simulink model "MCHP_SMO_MCLV48V300W_dsPIC33CK64MC105_DIM"  (R2022b)
settings: Solver=FixedStepDiscrete  StartTime=0.0  StopTime=10.0  FixedStep=50e-6  RelTol=1e-3  EnableMultiTasking=on
undefined symbols (not defined in the file): A4, B0, C12, C13, C4, C5, C6, C8, C9, DiscIntNeverNeededParam, inverter, Iq_Ref_openLoop, Max, MaxPer, ms, NumBits1, NumBits2, P20, P32, P52, P53, P54, P56, P57, P60, P61, PI_params, Pin, pmsm, PU_System, PWM1max, PWM_frequency, Resol, s, Speed_Ref_openLoop, Ts, Ts_speed, us
libraries: simulink x30, MCHP_Blockset x18, mcbcontrolslib x9, slpidlib x3, mcbplantlib x1, autolibpmsmexterior x1
(part 1 of 4)
settings Model: ExtModeBatchMode=on  ExtModeEnableFloating=off  ExtModeTrigDuration=32  Creator=I67977  LastModifiedBy=I67977
settings OptimizationCC: DefaultParameterBehavior=Inlined  DefaultUnderspecifiedDataType=single  InlineInvariantSignals=on  EnhancedBackFolding=on  StrengthReduction=on  BooleansAsBitfields=on  PassReuseOutputArgsAs=Individual arguments  ZeroExternalMemoryAtStartup=off  ZeroInternalMemoryAtStartup=off  OptimizeBlockOrder=speed  DifferentSizesBufferReuse=on  EfficientTunableParamExpr=on
settings DebuggingCC: MultiTaskDSMMsg=none  MultiTaskCondExecSysMsg=none  MultiTaskRateTransMsg=warning  ParameterTunabilityLossMsg=error
settings HardwareCC: ProdBitPerInt=16  ProdBitPerPointer=16  ProdBitPerSizeT=16  ProdBitPerPtrDiffT=32  ProdLargestAtomicInteger=Integer  ProdLargestAtomicFloat=None  ProdWordSize=16  ProdLongLongMode=on  ProdHWDeviceType=Generic->Custom
settings ModelReferenceCC: ModelReferenceNumInstancesAllowed=Single
settings SFSimCC: MATLABDynamicMemAlloc=off
settings RTWCC: Description=Microchip Embedded Target PIC24 dsPIC30 dsPIC33 (real-time)  SystemTargetFile=MCHP_dsPIC_stf.tlc  TLCOptions="-aExtModeXCPClassicInterface=0  -aCreateExtModeTypes=1 -aExtModeXCPSimulationTimeInTicks=1"  TemplateMakefile=MCHP_dsPIC.tmf
settings CodeAppCC: ForceParamTrailComments=on  IgnoreCustomStorageClasses=off  MaxIdLength=255  OperatorAnnotations=on  SimulinkDataObjDesc=on  SFDataObjDesc=on  InsertBlockDesc=on
settings STFCustomTargetCC: TargetLibSuffix=_lib.a  CodeReplacementLibrary=Microchip Code Replacement Library for dsPIC  MultiwordLength=256  CombineOutputUpdateFcns=on  CombineSignalStateStructs=on  SuppressErrorStatus=on  ERTCustomFileBanners=on  SupportNonFinite=off  SupportContinuousTime=off  RemoveResetFunc=on  MATLABClassNameForMDSCustomization=Simulink.SoftwareTarget.ERTCustomization  SystemTargetFile=MCHP_dsPIC_stf.tlc
settings ERTTargetCC: TargetLibSuffix=_lib.a  CodeReplacementLibrary=Microchip Code Replacement Library for dsPIC  ParMdlRefBuildCompliant=off  CompOptLevelCompliant=off  ConcurrentExecutionCompliant=off  CombineSignalStateStructs=on  SuppressErrorStatus=on  SupportNonFinite=off  SupportNonInlinedSFcns=on  ModelStepFunctionPrototypeControlCompliant=off  CPPClassGenCompliant=off  UseToolchainInfoCompliant=off  ExtModeTransport=1  ExtModeStaticAlloc=on  ExtModeAutomaticAllocSize=off  ExtModeStaticAllocSize=2048  ExtModeMexFile=ext_xcp  ExtModeMexArgs=1 0 4000000 './MCHP_LVMC_template.X/MCHP_LVMC_template.elf'  ExtModeIntrfLevel=Level2 - Open  InlinedParameterPlacement=NonHierarchical  ERTSrcFileBannerTemplate=MCHP_dsPIC_code_template.cgt  ERTHdrFileBannerTemplate=MCHP_dsPIC_code_template.cgt  ERTDataSrcFileTemplate=MCHP_dsPIC_code_template.cgt  ERTDataHdrFileTemplate=MCHP_dsPIC_code_template.cgt  ERTCustomFileTemplate=MCHP_main.tlc  MaxLineWidth=110

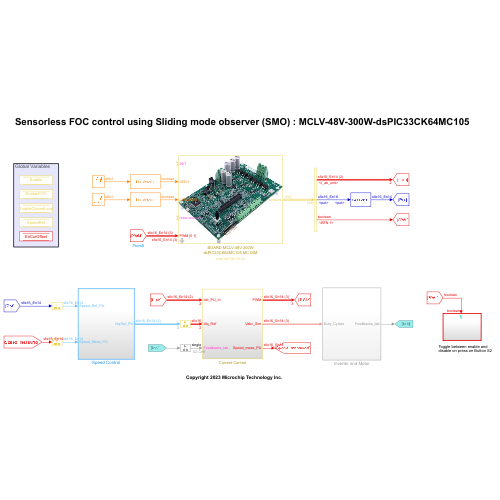
[thumbnail: Simulink's stored preview of the top-level diagram]
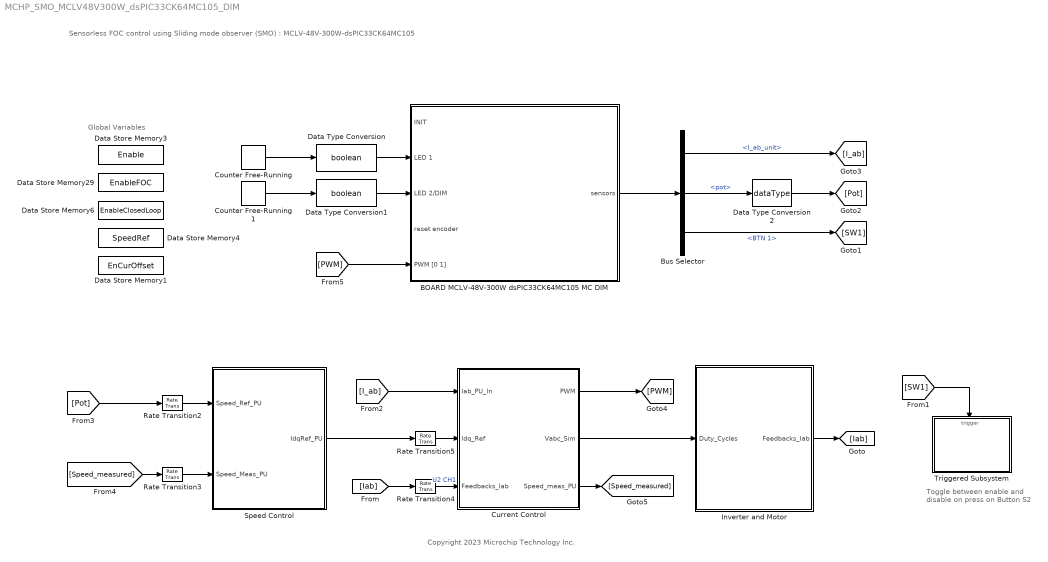
== system MCHP_SMO_MCLV48V300W_dsPIC33CK64MC105_DIM ==
  note: Toggle between enable and disable on press on Button S2
  note: Copyright 2023 Microchip Technology Inc.
  note: Global Variables
  note: Sensorless FOC control using Sliding mode observer (SMO) : MCLV-48V-300W-dsPIC33CK64MC105
  BOARD MCLV-48V-300W dsPIC33CK64MC105 MC DIM : Subsystem  mask(MCLV-48V-300W - dsPIC33CK64MC105 MC DIM using internal Op-Amp){boardVariants=internal Op-Amp, n=4, QEIResolution=4000, QEI_Reset=on index signal, QEI_Offset_settings=0, QEIOffset=0}
      mask prompts: boardVariants "board variants"; n "Motor poles pairs"; QEIResolution "Optical encoder resolution per mechanical rotation (lines)"; QEI_Reset "Optical encoder reset"; QEI_Offset_settings "Optical encoder offset (mechanical in rad)"; QEIOffset "Optical encoder offset (mechanical in rad)"
      mask help:
      | Template for motor control algorithm. Open subsystem (ctrl-u) for further customisation.
      |
      | Block bus output provices:
      |   - Current phase ia & ib, DC bus and potentiometer position
      |   - Buttons (0 when pressed, 1 for Btn 3 unconnected)
      |   - QEI position and velocity
      |   - MCU load and overload
      |
      | Block inputs:
      |   - INIT signal average the current phase ia and ib to be removed
      |   - LEDs
      |   - Reset encoder allows to align the motor while reseting the encoder
      |   - PWM normalized duty cycle value
      |
      | Model 50us base rate (20kHz) is synchronized with ADC conversion which is synchronized with the 50us PWM periods
      mask init:
      | BlksQEI = find_system(gcb,'FollowLinks','on','LookUnderMasks','all','ReferenceBlock','MCHP_Blockset/QEI/QEI');
      | QEI_Reset = get_param(gcb,'QEI_Reset');
      | if numel(BlksQEI) >= 1
      |     switch QEI_Reset
      |         case 'on index signal'
      |             set_param(BlksQEI{1},'PIMOD_mode','RESET position on each INDEX event');
      |         case 'on logical input (software)'        
      |             set_param(BlksQEI{1},'PIMOD_mode','position is cyclique between user defined boundaries'); 
      |         case 'custom setting'
      |             % do nothing 
      |     end
      | end % if
      | 
      |     BlksOpAmp = find_system(gcb,'FollowLinks','on','IncludeCommented','on','LookUnderMasks','all','ReferenceBlock','MCHP_Blockset/Analog IO/Op-Amp');
      |     if numel(BlksOpAmp) >= 1
      |         boardVariants = get_param(gcb,'boardVariants');
      |         switch boardVariants
      |             case 'internal Op-Amp'
      |                 set_param(BlksOpAmp{1},'Commented','off');
      |             case 'external Op-Amp'
      |                 set_param(BlksOpAmp{1},'Commented','on');
      |         end
      |     end % if
      settings: AttributesFormatString=%<boardVariants>
      mask TypeOptions boardVariants: internal Op-Amp | external Op-Amp
      mask TypeOptions n: 1 | 2 | 3 | 4 | 5 | 6 | 7 | 8 | 9 | 10 | 11 | 12 | 13 | 14 | 15 | 16
      mask TypeOptions QEI_Reset: on index signal | on logical input (software) | custom setting
      mask Callback QEI_Reset:
      | QEI_Reset = get_param(gcb,'QEI_Reset');
      | switch QEI_Reset
      |     case 'on index signal'
      |         QEIOffset = MCHP_Fun.Evalin('base','QEIOffset');
      |         set_param(gcb,'QEIOffset',num2str(QEIOffset));
      |         set_param(gcb,'MaskVisibilities',{'on';'on';'on';'on';'on';'off'});
      |     case 'on logical input (software)'
      |         set_param(gcb,'QEIOffset','0');
      |         set_param(gcb,'MaskVisibilities',{'on';'on';'on';'on';'off';'off'});
      |     case 'custom setting'
      |         set_param(gcb,'MaskVisibilities',{'on';'on';'on';'on';'on';'off'});
      |         % do nothing
      | end
      mask DialogControl n Tooltip: Number of pole pairs of the motor
      mask DialogControl QEIResolution Tooltip: encoder resolution per mechanical rotation
      mask DialogControl QEI_Reset Tooltip: enable encoder index signal if available. Otherwise align motor by applying a tension and set the rst input to 1
      mask DialogControl QEI_Offset_settings Tooltip: offset angle between encoder index and motor winding reference axis applied on theta_m and theta_e
      mask Display: image('$imagefile'); % Use "Edit Image" on toolstrip to change.
  Bus Selector : BusSelector  OutputSignals=ADC_unit.I_ab_unit,ADC.pot,BTN.BTN 1
  Counter Free-Running : simulink/Sources/Counter Free-Running  NumBits=1  tsamp=0.5
  Counter Free-Running1 : simulink/Sources/Counter Free-Running  NumBits=1  tsamp=0.1
  Current Control : Subsystem
  Data Store Memory1 : DataStoreMemory  DataStoreName=EnCurOffset  ShowAdditionalParam=off  OutDataTypeStr=boolean
  Data Store Memory29 : DataStoreMemory  DataStoreName=EnableFOC  ShowAdditionalParam=off  OutDataTypeStr=boolean
  Data Store Memory3 : DataStoreMemory  DataStoreName=Enable  ShowAdditionalParam=off  OutDataTypeStr=boolean
  Data Store Memory4 : DataStoreMemory  DataStoreName=SpeedRef  ShowAdditionalParam=off  OutDataTypeStr=dataType
  Data Store Memory6 : DataStoreMemory  DataStoreName=EnableClosedLoop  ShowAdditionalParam=off  OutDataTypeStr=boolean
  Data Type Conversion : DataTypeConversion  OutDataTypeStr=boolean  SaturateOnIntegerOverflow=off  RndMeth=Floor
  Data Type Conversion1 : DataTypeConversion  OutDataTypeStr=boolean  SaturateOnIntegerOverflow=off  RndMeth=Floor
  Data Type Conversion2 : DataTypeConversion  OutDataTypeStr=dataType  RndMeth=Simplest  SaturateOnIntegerOverflow=off
  Inverter and Motor : Subsystem
  Rate Transition{2..5} (4 alike) : RateTransition  Deterministic=off
  Speed Control : Subsystem  TreatAsAtomicUnit=on  SystemSampleTime=Ts_speed
  Triggered Subsystem : Subsystem  TreatAsAtomicUnit=on
  wires:
  [Iab] -> Rate Transition4/1
  Rate Transition4/1 -> Current Control/3(Feedbacks_Iab)  "U2 CH1"
  Current Control/2(Vabc_Sim) -> Inverter and Motor/1(Duty_Cycles)
  [Pot] -> Rate Transition2/1
  Rate Transition3/1 -> Speed Control/2(Speed_Meas_PU)
  [Speed_measured] -> Rate Transition3/1
  Rate Transition2/1 -> Speed Control/1(Speed_Ref_PU)
  Inverter and Motor/1(Feedbacks_Iab) -> [Iab]
  [I_ab] -> Current Control/1(Iab_PU_In)
  Rate Transition5/1 -> Current Control/2(Idq_Ref)
  Current Control/3(Speed_meas_PU) -> [Speed_measured]
  [SW1] -> Triggered Subsystem/Trigger
  Speed Control/1(IdqRef_PU) -> Rate Transition5/1
  Current Control/1(PWM) -> [PWM]
  Bus Selector/2 -> Data Type Conversion2/1  "<pot>"
  Bus Selector/3 -> [SW1]  "<BTN 1>"
  Bus Selector/1 -> [I_ab]  "<I_ab_unit>"
  Data Type Conversion2/1 -> [Pot]
  BOARD MCLV-48V-300W dsPIC33CK64MC105 MC DIM/1(sensors) -> Bus Selector/1
  Counter Free-Running/1 -> Data Type Conversion/1
  Counter Free-Running1/1 -> Data Type Conversion1/1
  Data Type Conversion/1 -> BOARD MCLV-48V-300W dsPIC33CK64MC105 MC DIM/2(LED 1)
  Data Type Conversion1/1 -> BOARD MCLV-48V-300W dsPIC33CK64MC105 MC DIM/3(LED 2/DIM)
  [PWM] -> BOARD MCLV-48V-300W dsPIC33CK64MC105 MC DIM/5(PWM [0 1])
